simulink model "AtrasoSim"  (R2015a)
settings: Solver=ode45  StartTime=0.0  StopTime=200  RelTol=1e-2
settings Model: Creator=user  LastModifiedBy=user

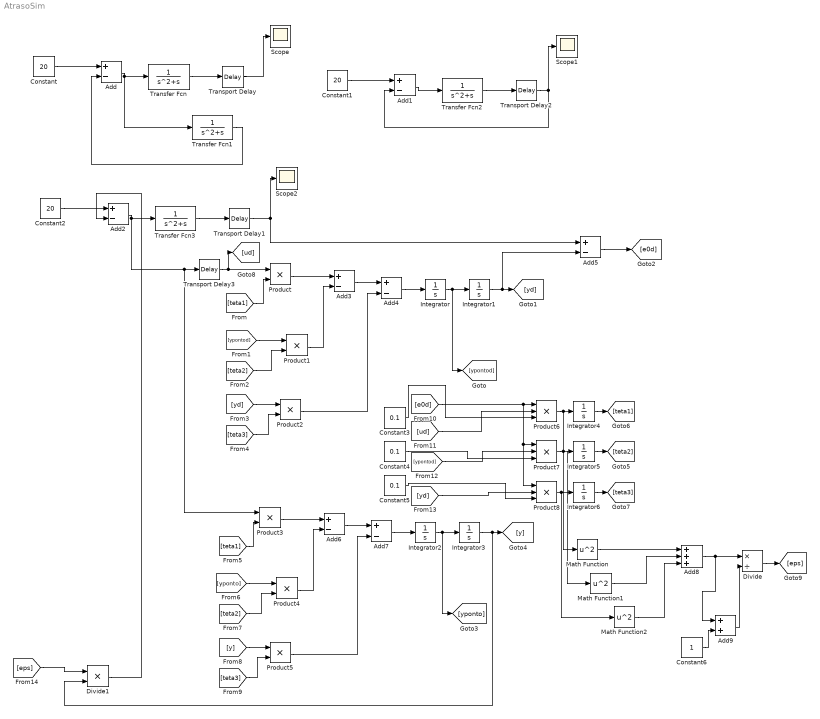
== system AtrasoSim ==
  Add{,1..7} (8 alike) : Sum  Inputs=+-
  Add8 : Sum  Inputs=+++
  Add9 : Sum
  Constant : Constant  Value=20
  Constant1 : Constant  Value=20
  Constant2 : Constant  Value=20
  Constant3 : Constant  Value=0.1
  Constant4 : Constant  Value=0.1
  Constant5 : Constant  Value=0.1
  Constant6 : Constant
  Divide : Product  Inputs=*/
  Divide1 : Product  Inputs=**
  Integrator{,1..6} (7 alike) : Integrator
  Math Function : Math  Operator=square  SaturateOnIntegerOverflow=on
  Math Function1 : Math  Operator=square  SaturateOnIntegerOverflow=on
  Math Function2 : Math  Operator=square  SaturateOnIntegerOverflow=on
  Product{,1..5} (6 alike) : Product
  Product6 : Product  Inputs=3
  Product7 : Product  Inputs=3
  Product8 : Product  Inputs=3
  Scope : Scope
  Scope1 : Scope
  Scope2 : Scope
      settings: SaveName=ScopeData2
  Transfer Fcn{,1..3} (4 alike) : TransferFcn  Denominator=[1 1 0]
  Transport Delay{,1..3} (4 alike) : TransportDelay  DelayTime=10
  wires:
  Transfer Fcn/1 -> Transport Delay/1
  Add/1 -> Transfer Fcn1/1, Transfer Fcn/1
  Transport Delay/1 -> Scope/1
  Transfer Fcn1/1 -> Add/2
  Constant/1 -> Add/1
  Transfer Fcn2/1 -> Transport Delay2/1
  Add1/1 -> Transfer Fcn2/1
  Constant1/1 -> Add1/1
  Transport Delay2/1 -> Add1/2, Scope1/1
  Transfer Fcn3/1 -> Transport Delay1/1
  Add2/1 -> Product3/1, Transport Delay3/1, Transfer Fcn3/1
  Transport Delay1/1 -> Add5/1, Scope2/1
  Integrator3/1 -> Divide1/2, [y]
  Constant2/1 -> Add2/1
  Transport Delay3/1 -> [ud], Product/1
  [teta1] -> Product/2
  Product/1 -> Add3/1
  Product1/1 -> Add3/2
  [ypontod] -> Product1/1
  [teta2] -> Product1/2
  [yd] -> Product2/1
  Add3/1 -> Add4/1
  Product2/1 -> Add4/2
  [teta3] -> Product2/2
  Add4/1 -> Integrator/1
  Integrator/1 -> [ypontod], Integrator1/1
  Integrator1/1 -> Add5/2, [yd]
  Add5/1 -> [e0d]
  [teta1] -> Product3/2
  Product4/1 -> Add6/2
  [yponto] -> Product4/1
  [teta2] -> Product4/2
  [y] -> Product5/1
  Product5/1 -> Add7/2
  [teta3] -> Product5/2
  Add7/1 -> Integrator2/1
  Integrator2/1 -> [yponto], Integrator3/1
  Product3/1 -> Add6/1
  Add6/1 -> Add7/1
  Product6/1 -> Math Function/1, Integrator4/1
  Integrator4/1 -> [teta1]
  Integrator5/1 -> [teta2]
  Integrator6/1 -> [teta3]
  [e0d] -> Product8/1, Product7/1, Product6/1
  Product7/1 -> Math Function1/1, Integrator5/1
  Product8/1 -> Math Function2/1, Integrator6/1
  [ud] -> Product6/2
  [ypontod] -> Product7/2
  [yd] -> Product8/2
  Constant3/1 -> Product6/3
  Constant4/1 -> Product7/3
  Constant5/1 -> Product8/3
  Math Function/1 -> Add8/1
  Math Function1/1 -> Add8/2
  Math Function2/1 -> Add8/3
  Add8/1 -> Add9/1, Divide/1
  Constant6/1 -> Add9/2
  Add9/1 -> Divide/2
  Divide/1 -> [eps]
  [eps] -> Divide1/1
  Divide1/1 -> Add2/2
